simulink model "Simulink_host"  (R2019b)
settings: Solver=FixedStepAuto  StartTime=0.0  StopTime=inf  RelTol=1e-3  EnableMultiTasking=on
libraries: legoev3lib x4
settings Model: ExtModeTrigDuration=2  Creator=nikit  LastModifiedBy=nikit
settings SolverCC: PositivePriorityOrder=on
settings OptimizationCC: EnhancedBackFolding=on  PassReuseOutputArgsAs=Individual arguments  ZeroExternalMemoryAtStartup=off  ZeroInternalMemoryAtStartup=off  MaxStackSize=64  OptimizeBlockOrder=speed  DifferentSizesBufferReuse=on  OptimizationCustomize=off  EfficientTunableParamExpr=on
settings DebuggingCC: ParameterTunabilityLossMsg=error
settings HardwareCC: ProdBitPerPointer=32  ProdBitPerSizeT=32  ProdBitPerPtrDiffT=32  ProdLargestAtomicInteger=Long  ProdWordSize=32  ProdHWDeviceType=ARM Compatible->ARM 9
settings SFSimCC: MATLABDynamicMemAlloc=off
settings RTWCC: SystemTargetFile=ert.tlc  HardwareBoard=LEGO MINDSTORMS EV3  TLCOptions="-aInlineSetEventsForThisBaseRateFcn=TLC_FALSE -aSuppressMultiTaskScheduler=TLC_FALSE  -aRateBasedStepFcn=0"  TemplateMakefile=ert_default_tmf  GenerateReport=on  Toolchain=Sourcery G++ Lite v2009q3  IncludeHyperlinkInReport=on  LaunchReport=on  GenerateTraceInfo=on  GenerateTraceReport=on  GenerateTraceReportSl=on  GenerateTraceReportSf=on  GenerateTraceReportEml=on
settings CodeAppCC: ForceParamTrailComments=on  IgnoreCustomStorageClasses=off  OperatorAnnotations=on  SimulinkDataObjDesc=on  SFDataObjDesc=on  InsertBlockDesc=on
settings ERTTargetCC: SupportContinuousTime=on  SupportVariableSizeSignals=on

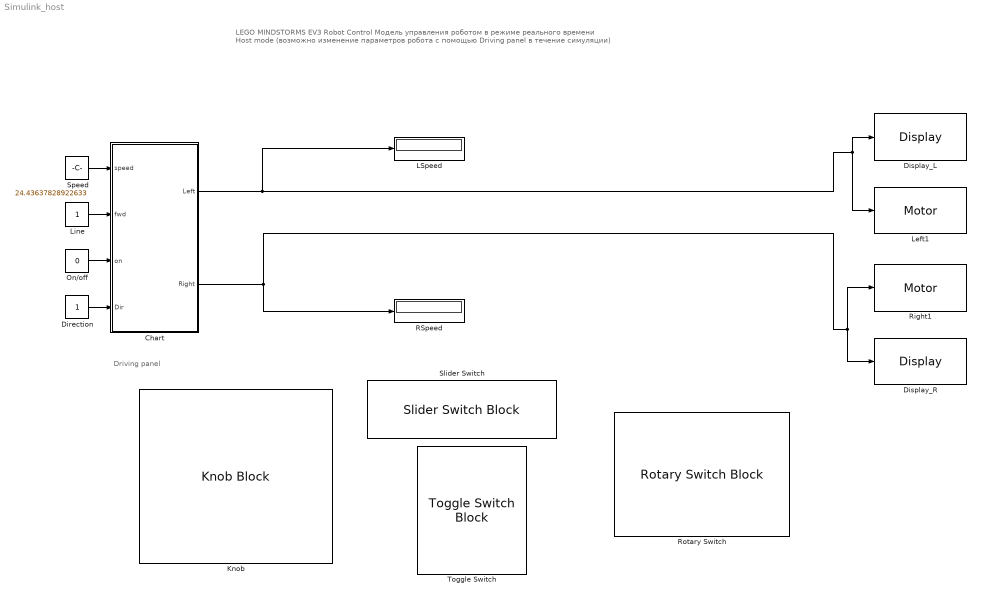
== system Simulink_host ==
  note: Driving panel
  note: LEGO MINDSTORMS EV3 Robot Control
      | Модель управления роботом в режиме реального времени Host mode
      | (возможно изменение параметров робота с помощью Driving panel в течение симуляции)
  Chart : Stateflow chart  TreatAsAtomicUnit=on
  Direction : Constant  OutDataTypeStr=int8
  Display_L : legoev3lib/Display  slcdStr=Left  slcdLine=1  slcdFormat=Decimal
      settings: SourceProductName=Simulink Support Package for LEGO MINDSTORMS EV3 Hardware  SourceProductBaseCode=LEGOEV3
  Display_R : legoev3lib/Display  slcdStr=Right  slcdLine=2  slcdFormat=Decimal
      settings: SourceProductName=Simulink Support Package for LEGO MINDSTORMS EV3 Hardware  SourceProductBaseCode=LEGOEV3
  Knob : KnobBlock
  LSpeed : Display
  Left1 : legoev3lib/Motor  sportNumber=A  sstopAction=Brake
  Line : Constant  OutDataTypeStr=int8
  On/off : Constant  Value=0  OutDataTypeStr=int8
  RSpeed : Display
  Right1 : legoev3lib/Motor  sportNumber=D  sstopAction=Brake
  Rotary Switch : RotarySwitchBlock
      settings: Values={{'Left', 'Forward', 'Right'}, [1 2 3]}
  Slider Switch : SliderSwitchBlock
      settings: Values={{'Off', 'On'}, [0 1]}
  Speed : Constant  Value=24.43637828922633  OutDataTypeStr=int8
  Toggle Switch : ToggleSwitchBlock
      settings: Values={{'Back', 'Forward'}, [-1 1]}
  wires:
  Chart/1(Left) -> Left1/1, Display_L/1, LSpeed/1
  Chart/2(Right) -> Display_R/1, Right1/1, RSpeed/1
  Line/1 -> Chart/2(fwd)
  Speed/1 -> Chart/1(speed)
  On/off/1 -> Chart/3(on)
  Direction/1 -> Chart/4(Dir)

== stateflow chart Simulink_host/Chart ==
  state Straight
    during:
    Left = speed*fwd*on;
    Right = Left;
  state Left_Diagonal
    during:
    Right = speed*fwd*on;
    Left = 0.5*Right;
  state Right_Diagonal
    during:
    Left = speed*fwd*on;
    Right = 0.5*Left;
  Right_Diagonal -> Left_Diagonal [order 2] : [Dir ==1]
  Left_Diagonal -> Right_Diagonal [order 2] : [Dir ==3]
  (default) -> Straight
  Straight -> Left_Diagonal [order 1] : [Dir ==1]
  Left_Diagonal -> Straight [order 1] : [Dir ==2]
  Right_Diagonal -> Straight [order 1] : [Dir ==2]
  Straight -> Right_Diagonal [order 2] : [Dir ==3]
  data: Left output int8 size=1; speed input int8; fwd input int8; on input int8; Dir input int8; Right output int8
